simulink model "atthw10p4"  (R2018b)
settings: Solver=VariableStepAuto  StartTime=0.0  StopTime=6000  RelTol=1e-3
settings Model: Creator=Eric  LastModifiedBy=Eric

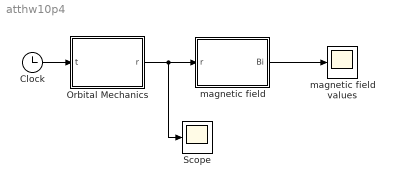
== system atthw10p4 ==
  Clock : Clock
  Orbital Mechanics : MATLAB Function  TreatAsAtomicUnit=on
  Scope : Scope
  magnetic field : MATLAB Function  TreatAsAtomicUnit=on
  magnetic field values : Scope
  wires:
  Clock/1 -> Orbital Mechanics/1(t)
  magnetic field/1(Bi) -> magnetic field values/1
  Orbital Mechanics/1(r) -> Scope/1, magnetic field/1(r)

== matlab function atthw10p4/Orbital Mechanics ==
  data: t input; r output
function r  = fcn(t)
mu = 398600.4415;
rho = 6600; %km

w = sqrt(mu/rho^3);
r = (rho/sqrt(2))*[-cos(w*t); sqrt(2)*sin(w*t); cos(w*t)];

== matlab function atthw10p4/magnetic field ==
  data: r input; Bi output
function Bi = fcn(r)

Bo = 3.12E-5;
Re = 6371; %km

%DCM inertial to NEZ;
nz = -r/norm(r);
ny = (cross(nz, [0; 0; 1]))/norm(cross(nz, [0; 0; 1]));
nx = cross(ny, nz);

Ti2ned = [ nx'; ny'; nz'];


lambda = asin(r(1)/norm(r));
%magnetic field calculation
Bn = Bo*((Re/norm(r))^3)*[cos(lambda); 0; -2*cos(lambda)];
Bi = Ti2ned'*Bn;
